simulink model "r_hw_31"  (R2019a)
settings: Solver=VariableStepAuto  StartTime=0.0  StopTime=10.0  RelTol=1e-3
libraries: simulink x1
settings Model: Creator=Tamer  LastModifiedBy=Tamer

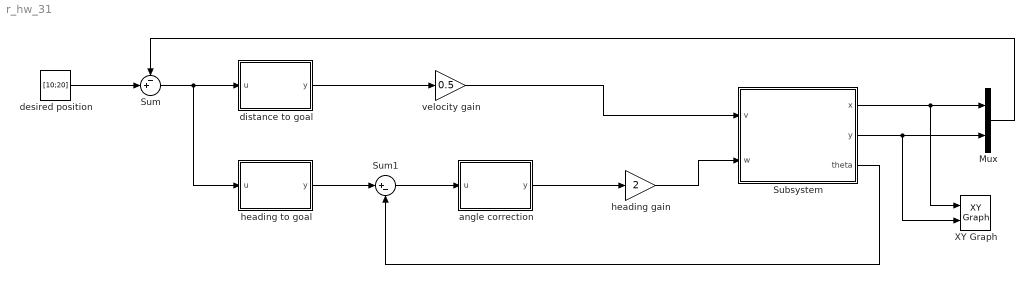
== system r_hw_31 ==
  Mux : Mux  Inputs=2
  Subsystem : Subsystem
  Sum : Sum  Inputs=-+|
  Sum1 : Sum  Inputs=|+-
  XY Graph : simulink/Sinks/XY Graph  xmin=-1  xmax=12  ymin=-1  ymax=22  st=-1
  angle correction : MATLAB Function  TreatAsAtomicUnit=on
  desired position : Constant  Value=[10;20]
  distance to goal : MATLAB Function  TreatAsAtomicUnit=on
  heading gain : Gain  Gain=2
  heading to goal : MATLAB Function  TreatAsAtomicUnit=on
  velocity gain : Gain  Gain=0.5
  wires:
  desired position/1 -> Sum/2
  Sum/1 -> heading to goal/1(u), distance to goal/1(u)
  distance to goal/1(y) -> velocity gain/1
  heading to goal/1(y) -> Sum1/1
  Sum1/1 -> angle correction/1(u)
  angle correction/1(y) -> heading gain/1
  Subsystem/1(x) -> XY Graph/1, Mux/1
  Subsystem/2(y) -> XY Graph/2, Mux/2
  heading gain/1 -> Subsystem/2(w)
  velocity gain/1 -> Subsystem/1(v)
  Subsystem/3(theta) -> Sum1/2
  Mux/1 -> Sum/1

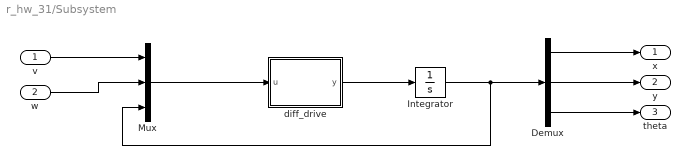
== system r_hw_31/Subsystem ==
  v : Inport
  w : Inport  Port=2
  Demux : Demux  Outputs=3
  Integrator : Integrator  InitialCondition=[0;0;0]
  Mux : Mux  Inputs=3
  diff_drive : MATLAB Function  TreatAsAtomicUnit=on
  x : Outport
  y : Outport  Port=2
  theta : Outport  Port=3
  wires:
  v/1 -> Mux/1
  w/1 -> Mux/2
  Mux/1 -> diff_drive/1(u)
  diff_drive/1(y) -> Integrator/1
  Integrator/1 -> Mux/3, Demux/1
  Demux/1 -> x/1
  Demux/2 -> y/1
  Demux/3 -> theta/1

== matlab function r_hw_31/heading to goal ==
  data: u input; y output
function y = fcn(u)
%u(1) : x' - x
%u(2) : y' - y
y = atan2(u(2),u(1));

== matlab function r_hw_31/distance to goal ==
  data: u input; y output
function y = fcn(u)
%u(1) : x' - x
%u(2) : y' - y
y = sqrt(u(1)^2+u(2)^2);

== matlab function r_hw_31/angle correction ==
  data: u input; y output
function y = fcn(u)
%u(1) : theta* - theta
y = atan2(sin(u(1)),cos(u(1)));

== matlab function r_hw_31/Subsystem/diff_drive ==
  data: u input; y output
function y = fcn(u)
%u(1) : v
%u(2) : w
%u(3) : x
%u(4) : y
%u(5) : phi

y = [u(1)*cos(u(5)); u(1)*sin(u(5));u(2)];
